simulink model "Teach_Points"  (Simulink 10.1)
settings: Solver=ode1  StartTime=0.0  StopTime=inf  FixedStep=0.01  RelTol=1e-3  EnableMultiTasking=on
libraries: quarc_library x1
settings Model: Creator=RSamra  LastModifiedBy=USER  SimulationMode=external  ExtModeTrigDuration=5000
settings SolverCC: PositivePriorityOrder=on
settings DataIOCC: LimitDataPoints=on  SignalLoggingSaveFormat=ModelDataLogs
settings OptimizationCC: ExpressionDepthLimit=2147483647  InitFltsAndDblsToZero=on
settings DebuggingCC: SolverPrmCheckMsg=warning  FcnCallInpInsideContextMsg=warning  StateNameClashWarn=warning
settings SFSimCC: SimParseCustomCode=off
settings RTWCC: Description=QUARC Win64 Target  SystemTargetFile=quarc_win64.tlc  TemplateMakefile=quarc_default_tmf
settings STFCustomTargetCC: TargetPreCompLibLocation=C:\PROGRA~3\QUARC\lib\2020a\win64\release  ConcurrentExecutionCompliant=on  CombineOutputUpdateFcns=on  CPPClassGenCompliant=on  GRTInterface=off  SystemTargetFile=quarc_win64.tlc
settings GRTTargetCC: TargetPreCompLibLocation=C:\PROGRA~3\QUARC\lib\2020a\win64\release  ParMdlRefBuildCompliant=off  CompOptLevelCompliant=off  CombineOutputUpdateFcns=on  MatFileLogging=off  GRTInterface=off  UseToolchainInfoCompliant=off  ExtMode=on  ExtModeMexFile=quarc_comm

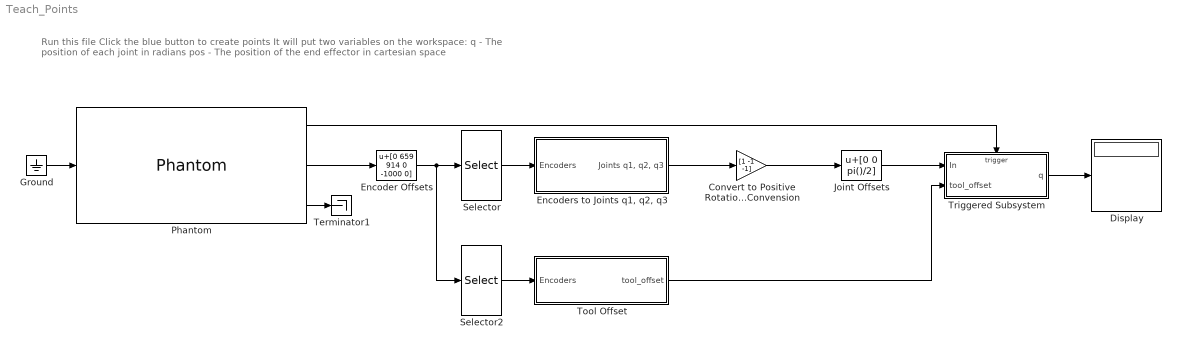
== system Teach_Points ==
  note: Run this file
      | Click the blue button to create points
      | It will put two variables on the workspace: q - The position of each joint in radians
      |                                                                  pos - The position of the end effector in cartesian space
  Convert to Positive Rotation Convension : Gain  Gain=[1 -1 -1]
  Display : Display
  Encoder Offsets : Bias  Bias=[0 659 914 0 -1000 0]
  "Encoders to Joints q1, q2, q3" : Subsystem
  Ground : Ground
  Joint Offsets : Bias  Bias=[0 0 pi()/2]
  Phantom : quarc_library/Devices/Third-Party/SensAble/Phantom/Phantom  device_name=Default Device  output_type=Encoders Values  input_type=Joint space  velocity_limit_option=on  velocity_limit=1200  is_7dof=off  sample_time=-1
      settings: AttributesFormatString=(%<device_name>)  SourceProductName=QUARC Targets
  Selector : Selector  InputPortWidth=6  IndexOptions=Index vector (dialog)  Indices=[1:3]  OutputSizes=1
  Selector2 : Selector  InputPortWidth=6  IndexOptions=Index vector (dialog)  Indices=[4:6]  OutputSizes=1
  Terminator1 : Terminator
  Tool Offset : MATLAB Function  TreatAsAtomicUnit=on
  Triggered Subsystem : Subsystem  TreatAsAtomicUnit=on
  wires:
  Triggered Subsystem/1(q) -> Display/1
  "Encoders to Joints q1, q2, q3"/1("Joints q1, q2, q3") -> Convert to Positive Rotation Convension/1
  Convert to Positive Rotation Convension/1 -> Joint Offsets/1
  Joint Offsets/1 -> Triggered Subsystem/1(In)
  Phantom/1 -> Triggered Subsystem/Trigger
  Ground/1 -> Phantom/1
  Phantom/3 -> Terminator1/1
  Phantom/2 -> Encoder Offsets/1
  Encoder Offsets/1 -> Selector/1, Selector2/1
  Selector/1 -> "Encoders to Joints q1, q2, q3"/1(Encoders)
  Selector2/1 -> Tool Offset/1(Encoders)
  Tool Offset/1(tool_offset) -> Triggered Subsystem/2(tool_offset)

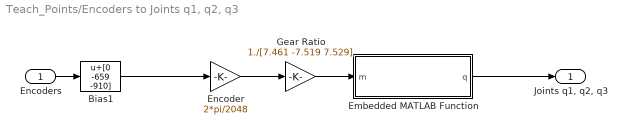
== system Teach_Points/Encoders to Joints q1, q2, q3 ==
  Encoders : Inport
  Bias1 : Bias  Bias=[0 -659 -910]
  Embedded MATLAB Function : MATLAB Function  TreatAsAtomicUnit=on
  Encoder : Gain  Gain=2*pi/2048
  Gear Ratio : Gain  Gain=1./[7.461 -7.519 7.529]
  "Joints q1, q2, q3" : Outport
  wires:
  Embedded MATLAB Function/1(q) -> "Joints q1, q2, q3"/1
  Encoders/1 -> Bias1/1
  Encoder/1 -> Gear Ratio/1
  Gear Ratio/1 -> Embedded MATLAB Function/1(m)
  Bias1/1 -> Encoder/1

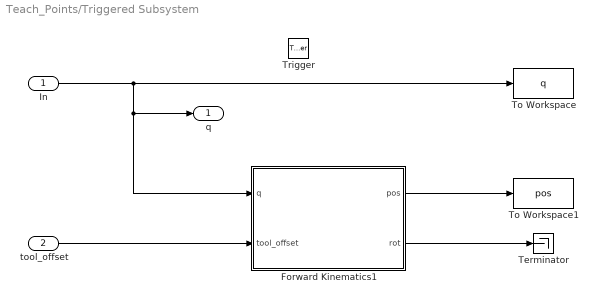
== system Teach_Points/Triggered Subsystem ==
  In : Inport
  tool_offset : Inport  Port=2
  Trigger : TriggerPort  VariantControl=(inherit)
  Forward Kinematics1 : MATLAB Function  TreatAsAtomicUnit=on
  Terminator : Terminator
  To Workspace : ToWorkspace  VariableName=q  SampleTime=-1
  To Workspace1 : ToWorkspace  VariableName=pos  SampleTime=-1
  q : Outport
  wires:
  In/1 -> To Workspace/1, q/1, Forward Kinematics1/1(q)
  tool_offset/1 -> Forward Kinematics1/2(tool_offset)
  Forward Kinematics1/1(pos) -> To Workspace1/1
  Forward Kinematics1/2(rot) -> Terminator/1

== matlab function Tool Offset ==
  data: Encoders input double; tool_offset output double
function tool_offset = getToolOffset(Encoders)

%convert encoder values to angles using bias and gain
bias = [-2048 -2654 -2048];
gain = [2*pi()/4915 2*pi()/4096 2*pi()/4915];
Angle = (Encoders' + bias).*gain;

% convert the angle to the positive rotation convention defined
% by DH parameters
pos_rot = [-1 1 1];
joint_offset = [0 -(40-180)*pi/180 0];
Joint456 = Angle.*pos_rot + joint_offset;

%pick off theta4 and theta5
theta4 = Joint456(1);
theta5 = Joint456(2);

% The orientation of the tool offset matrix is given two successive
% rotations about x and z axis. 
RotZ = [cos(theta5) -sin(theta5) 0; sin(theta5) cos(theta5) 0; 0 0 1];
RotX = [1 0 0; 0 cos(theta4) -sin(theta4); 0 sin(theta4) cos(theta4)];
R = RotX*RotZ; % R is the rotation matrix of the tool offset matrix with respect to frame 3

% with respect to frame 3, the tool is 0.039m in the x-direction. Convert
% this vector to tool frame coordinates
tool_pos =R * [.039; 0; 0];

%create a Tool_offset transformation matrix. Use Identity matrix for
%rotation to show that the end effector frame and frame 3 are always
%aligned
I = [1 0 0; 0 1 0; 0 0 1];
tool = cat(2,I,tool_pos);
tool_offset = cat(1,tool,[0 0 0 1]);

== matlab function Encoders to Joints q1, q2, q3/Embedded MATLAB Function ==
  data: m input double; q output double
function q = Motors_2_Joints(m)
q = m;
q(1) = m(1);
q(2) = m(2);
q(3) = m(3) - m(2) -pi/2;
end

== matlab function Triggered Subsystem/Forward Kinematics1 ==
  data: pos output double; q input double; rot output double; tool_offset input double
function [pos,rot]    = ForwardKinematics(q,tool_offset)
% This block supports the Embedded MATLAB subset.
% See the help menu for details. 

% Link lengths
L1 = .132;
L2 = .132;

%Define A-matrices
%A1= DH(theta ,d ,a ,alpha)
A1 = DH(q(1), 0, 0, -pi()/2);
A2 = DH(q(2), 0, L1, 0);
A3 = DH(q(3)-pi/2, 0, L2, 0);

%Define T Matrices
T01=A1;
T02=T01*A2;
T03=T02*A3;

%tool_offset given with respect to frame 3.
T_tool=T03*tool_offset;
rot=T_tool(1:3,1:3);
pos=T_tool(1:3,4);


end

function A = DH(theta, d, a, alpha)

A_R_z = [cos(theta) -sin(theta) 0 0;
         sin(theta) cos(theta) 0 0;
         0 0 1 0;
         0 0 0 1];

A_T_z = [1 0 0 0;
         0 1 0 0;
         0 0 1 d;
         0 0 0 1];
     
  

A_T_x = [1 0 0 a;
         0 1 0 0;
         0 0 1 0;
         0 0 0 1];

A_R_x = [1 0 0 0;
         0 cos(alpha) -sin(alpha)  0;
         0 sin(alpha) cos(alpha) 0;
         0 0 0 1];

A = A_R_z*A_T_z*A_T_x*A_R_x;

end
